simulink model "IO_test"  (R2022b)
settings: Solver=FixedStepAuto  StartTime=0.0  StopTime=10.0  FixedStep=0.1  RelTol=1e-3  EnableMultiTasking=on
libraries: bbblueBasicLib x1
settings Model: ExtModeTrigDuration=100  Creator=Nick  LastModifiedBy=Nick
settings SolverCC: PositivePriorityOrder=on
settings OptimizationCC: EnhancedBackFolding=on  PassReuseOutputArgsAs=Individual arguments  ZeroExternalMemoryAtStartup=off  ZeroInternalMemoryAtStartup=off  MaxStackSize=64  OptimizeBlockOrder=speed  DifferentSizesBufferReuse=on  OptimizationCustomize=off  EfficientTunableParamExpr=on
settings DebuggingCC: ParameterTunabilityLossMsg=error
settings HardwareCC: ProdBitPerPointer=32  ProdBitPerSizeT=32  ProdBitPerPtrDiffT=32  ProdLargestAtomicInteger=Long  ProdLargestAtomicFloat=Double  ProdWordSize=32  ProdHWDeviceType=ARM Compatible->ARM Cortex  UseEmbeddedCoderFeatures=off
settings SFSimCC: SimCustomHeaderCode="#include \"print_input.h\""  SimUserSources=C:\Users\Nick\Documents\Github\beaglebone-epos-can\simulink\placeholders\print_input.c  SimUserIncludeDirs=C:\Users\Nick\Documents\Github\beaglebone-epos-can\simulink\placeholders  MATLABDynamicMemAlloc=off
settings RTWCC: Description=Embedded Coder  SystemTargetFile=ert.tlc  HardwareBoard=BeagleBone Blue  TLCOptions="-aInlineSetEventsForThisBaseRateFcn=TLC_FALSE -aSuppressMultiTaskScheduler=TLC_FALSE  -aRateBasedStepFcn=0"  TemplateMakefile=ert_default_tmf  RTWUseSimCustomCode=on  CustomHeaderCode="#include \"print_input.h\""  CustomInclude=C:\Users\Nick\Documents\Github\beaglebone-epos-can\simulink\placeholders  CustomSource=C:\Users\Nick\Documents\Github\beaglebone-epos-can\simulink\placeholders\print_input.c  Toolchain=GNU GCC BeagleBone Blue
settings CodeAppCC: ForceParamTrailComments=on  IgnoreCustomStorageClasses=off  OperatorAnnotations=on  SimulinkDataObjDesc=on  SFDataObjDesc=on  InsertBlockDesc=on
settings ERTTargetCC: SupportNonInlinedSFcns=on  SupportVariableSizeSignals=on

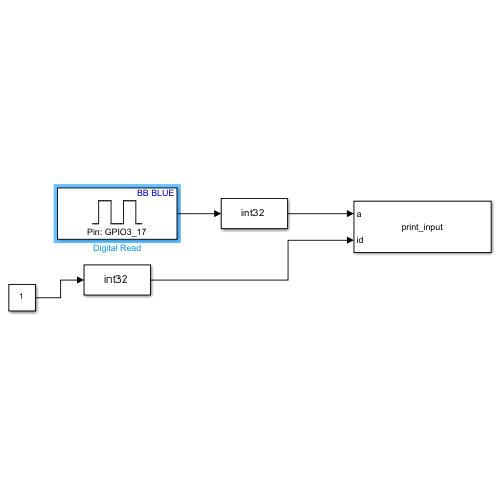
[thumbnail: Simulink's stored preview of the top-level diagram]
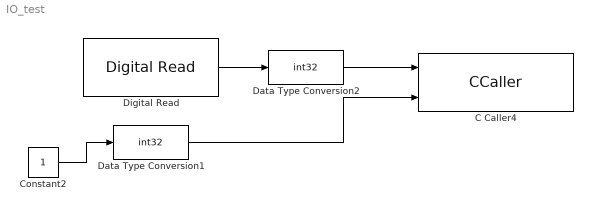
== system IO_test ==
  C Caller4 : CCaller  FunctionName=print_input  PortSpecificationStruct="%)30     .    N ,   8    (     @         %    \"     (    !     0         %  0 \"0    $    _    07)G3F%M90  4&]R=$YA;64 4V-O<&4     26YD97@     5'EP90      4VEZ90      27-';&]B86P   X    P    !@    @    $          4    (     0    $    !         !   0!A    #@   #     &    \"     0         !0    @    !     0    $         $  ! &$    .    .     8    (    !          %    \"     $    %     0         0    !0   $EN<'5T    #@   #@    &    \"     8         !0    @    !     0    $         \"0    @               X    X    !@    @    $          4    (     0    4    !         !     %    :6YT,S(    .    ,     8    (    !          %    \"     $    !     0         0  $ ,0    X    P    !@    @    ) @        4    (     0    $    !          (  0      #@   #     &    \"     0         !0    @    !     @    $         $  \" &ED   .    ,     8    (    !          %    \"     $    \"     0         0  ( :60   X    X    !@    @    $          4    (     0    4    !         !     %    26YP=70    .    .     8    (    !@         %    \"     $    !     0         )    \"            / _#@   #@    &    \"     0         !0    @    !    !0    $         $     4   !I;G0S,@    X    P    !@    @    $          4    (     0    $    !         !   0 Q    #@   #     &    \"     D\"        !0    @    !     0    $          @ !"  SampleTime=0.1
  Constant2 : Constant
  Data Type Conversion1 : DataTypeConversion  OutDataTypeStr=int32  SaturateOnIntegerOverflow=off  RndMeth=Floor
  Data Type Conversion2 : DataTypeConversion  OutDataTypeStr=int32  SaturateOnIntegerOverflow=off  RndMeth=Floor
  Digital Read : bbblueBasicLib/Digital Read  Pin=49  Direction=input  GPIOSelect=GPIO3_17  SampleTime=0.1
  wires:
  Digital Read/1 -> Data Type Conversion2/1
  Constant2/1 -> Data Type Conversion1/1
  Data Type Conversion1/1 -> C Caller4/2
  Data Type Conversion2/1 -> C Caller4/1
